simulink model "P2PHVDCMMC"  (R2024a)
settings: Solver=FixedStepDiscrete  StartTime=0.0  StopTime=10  RelTol=1e-3
PreLoadFcn:
  | % HVDCMMCInterconnectionParam
StartFcn:
  | tic
StopFcn:
  | toc
values from neighbouring files (symbols this model uses):
  C_PM = 1.758e-3    (= 0.001758)    [P2PHVDCMMCcode.m]    (also in SFu.mat)
  Cg = 50e-9    (= 5e-08)    [P2PHVDCMMCcode.m]    (also in SFu.mat)
  Fc = Fnom*3.37    (= 168.5)    [P2PHVDCMMCcode.m]    (also in SFu.mat)
  Fnom = 50    [P2PHVDCMMCcode.m]    (also in SFu.mat)
  HRM = 1    [SFu.mat]
  Ki_Ireg = 6    [P2PHVDCMMCcode.m]    (also in SFu.mat)
  Ki_Preg = 1.0    (= 1)    [P2PHVDCMMCcode.m]    (also in SFu.mat)
  Ki_Qreg = 1.0    (= 1)    [P2PHVDCMMCcode.m]    (also in SFu.mat)
  Ki_VDCreg = 100    [P2PHVDCMMCcode.m]    (also in SFu.mat)
  Kp_Ireg = 0.6    [P2PHVDCMMCcode.m]    (also in SFu.mat)
  Kp_Preg = 0.5/3    (= 0.166666666667)    [P2PHVDCMMCcode.m]    (also in SFu.mat)
  Kp_Qreg = 0.5/3    (= 0.166666666667)    [P2PHVDCMMCcode.m]    (also in SFu.mat)
  Kp_VDCreg = 4    [P2PHVDCMMCcode.m]    (also in SFu.mat)
  L_cable = 15e-3    (= 0.015)    [P2PHVDCMMCcode.m]    (also in SFu.mat)
  Larm = Larm_pu*(Zb_ac/(2*pi*Fnom))    [P2PHVDCMMCcode.m]    (also in SFu.mat = 0.0529455974536)
  Larm_pu = 0.15    [P2PHVDCMMCcode.m]    (also in SFu.mat)
  Lff = Larm_pu/2    (= 0.075)    [P2PHVDCMMCcode.m]    (also in SFu.mat)
  Limits_Ireg = [ 2.0  -2.0]    [P2PHVDCMMCcode.m]    (also in SFu.mat = [2 -2])
  Limits_Preg = [ 1.2, 0.8 ]    [P2PHVDCMMCcode.m]    (also in SFu.mat = [1.2 0.8])
  Limits_Qreg = [ 0.25, -0.25 ]    [P2PHVDCMMCcode.m]    (also in SFu.mat = [0.25 -0.25])
  Limits_VDCreg = [ 2.0  -2.0]    [P2PHVDCMMCcode.m]    (also in SFu.mat = [2 -2])
  Lxfo = 0.12    [P2PHVDCMMCcode.m]    (also in SFu.mat)
  N = 1    [P2PHVDCMMCcode.m]    (also in SFu.mat)
  Nb_PM = 36    [P2PHVDCMMCcode.m]    (also in SFu.mat)
  Pnom = 1000e6    (= 1000000000)    [P2PHVDCMMCcode.m]    (also in SFu.mat)
  R_cable = 0.5    [P2PHVDCMMCcode.m]    (also in SFu.mat)
  R_startup = 400    [P2PHVDCMMCcode.m]    (also in SFu.mat)
  Rarm = Rarm_pu*Zb_ac    [P2PHVDCMMCcode.m]    (also in SFu.mat = 0.1663335)
  Rff = Rarm_pu/2    (= 0.00075)    [P2PHVDCMMCcode.m]    (also in SFu.mat)
  Rg = 100    [P2PHVDCMMCcode.m]    (also in SFu.mat)
  Rxfo = 0.003    [P2PHVDCMMCcode.m]    (also in SFu.mat)
  S =     [SFu.mat]
  Slope_Qref = 0.5    [P2PHVDCMMCcode.m]    (also in SFu.mat)
  Slope_Vdc_ref = Vnom_dc/5    (= 128000)    [P2PHVDCMMCcode.m]    (also in SFu.mat)
  Tfault = 9999    [SFu.mat]
  Ts = Ts_Control    (= 4e-05)    [P2PHVDCMMCcode.m]    (also in SFu.mat)
  Ts_Control = 40e-6    (= 4e-05)    [P2PHVDCMMCcode.m]    (also in SFu.mat)
  Ts_dqn = 2e-5    (= 2e-05)    [P2PHVDCMMCcode.m]    (also in SFu.mat)
  Ts_Power = 20e-6    (= 2e-05)    [P2PHVDCMMCcode.m]    (also in SFu.mat)
  Vnom_dc = 640e3    (= 640000)    [P2PHVDCMMCcode.m]    (also in SFu.mat)
  Vnom_prim = 400e3    (= 400000)    [P2PHVDCMMCcode.m]    (also in SFu.mat)
  Vnom_sec = 333e3    (= 333000)    [P2PHVDCMMCcode.m]    (also in SFu.mat)
  Ws = 314.159265359    [SFu.mat]
undefined symbols (not defined in the file or in its folder): DiscIntNeverNeededParam, Discrete, DQN_Lib, gcbh, Int_DQNc_Mat, Mult_DQNc_Mat, Pcc, sps, sps_rtmsupport, spsMeanValueVariableFrequencyModel, spsPLL3phModel, SY3
libraries: simulink x38, spsControlledVoltageSourceLib x30, spsVoltageMeasurementLib x21, spsIdealSwitchLib x21, powerlib_extras x12, spsSecondOrderFilterLib x12, spsCurrentMeasurementLib x12, spsdq0toabcLib x9, spsMeanLib x8, spsMeanVariableFrequencyLib x8, spsabctodq0Lib x8, spsThreePhaseSeriesRLCBranchLib x7
(part 4 of 13)

== system P2PHVDCMMC/Controllers3/PLL, Measurements and Transformation ==
  note: P (pu) = Vd*Id + Vq*Iq
  note: Q (pu) = Vq*Id - Vd*Iq
  note: P positive = Converter generates active power (Inverter Mode)
  note: Q positive = Converter generates reactive power (Capacitive Mode)
  Vabc : Inport  PortDimensions=3
  Iabc : Inport  Port=2  PortDimensions=3
  Add : Sum  Inputs=1
  Demux : Demux  Outputs=2
  Discrete Mean value : powerlib_extras/Discrete Measurements/Discrete  Mean value  Freq=Fnom  Vinit=0  Ts=Ts
  Discrete Mean value1 : powerlib_extras/Discrete Measurements/Discrete  Mean value  Freq=Fnom  Vinit=0  Ts=Ts
  I->pu2 : Gain  Gain=sqrt(3)*Vnom_sec/sqrt(2)/Pnom  SaturateOnIntegerOverflow=on  OutDataTypeStr=Inherit: Same as input  ParamDataTypeStr=Inherit: Same as input
  PLL (3ph) : spsPLL3phLib/PLL (3ph)  Fmin=0.9*Fnom  Par_Init=[0, Fnom]  ParK=[180, 3200, 1]  TcD=1e-4  MaxRateChangeFreq=12  FilterCutOffFreq=25  Ts=Ts  AGC=on
  Product : Product  RndMeth=Zero
  Product1 : Product  RndMeth=Zero
  Second-Order Filter : spsSecondOrderFilterLib/Second-Order Filter  FilterType=Lowpass  Fo=Fn_filter  Zeta=Zeta_filter  Ts=Ts  Initialize=off  Vac_Init="[0,  0,  60]"  Vdc_Init=0  PlotResponse=off  FreqRange=[0, 500, 1]
  Second-Order Filter1 : spsSecondOrderFilterLib/Second-Order Filter  FilterType=Lowpass  Fo=Fn_filter  Zeta=Zeta_filter  Ts=Ts  Initialize=off  Vac_Init="[0,  0,  60]"  Vdc_Init=0  PlotResponse=off  FreqRange=[0, 500, 1]
  Selector3 : Selector  InputPortWidth=2  IndexOptions=Index vector (dialog)  Indices=[2 1]  OutputSizes=1
  Selector4 : Selector  InputPortWidth=3  IndexOptions=Index vector (dialog)  Indices=[1 2]  OutputSizes=1
  Selector5 : Selector  InputPortWidth=3  IndexOptions=Index vector (dialog)  Indices=[1 2]  OutputSizes=1
  Subtract : Sum  Inputs=+-
  V->pu1 : Gain  Gain=1/(Vnom_sec/sqrt(3)*sqrt(2))  SaturateOnIntegerOverflow=on  OutDataTypeStr=Inherit: Same as input  ParamDataTypeStr=Inherit: Same as input
  abc to dq0 : spsabctodq0Lib/abc to dq0  Alignment=90 degrees behind phase A axis
  abc to dq1 : spsabctodq0Lib/abc to dq0  Alignment=90 degrees behind phase A axis
  Freq : Outport
  wt : Outport  Port=2
  VdVq : Outport  Port=3
  IdIq : Outport  Port=4
  P : Outport  Port=5
  Q : Outport  Port=6
  wires:
  Selector3/1 -> Product1/1
  Discrete Mean value1/1 -> Q/1
  Discrete Mean value/1 -> P/1
  Second-Order Filter/1 -> VdVq/1, Product/1, Selector3/1
  Second-Order Filter1/1 -> IdIq/1, Product1/2, Product/2
  Product/1 -> Add/1
  Product1/1 -> Demux/1
  Demux/1 -> Subtract/1
  Demux/2 -> Subtract/2
  Add/1 -> Discrete Mean value/1
  Subtract/1 -> Discrete Mean value1/1
  abc to dq0/1 -> Selector4/1
  PLL (3ph)/1 -> Freq/1
  V->pu1/1 -> abc to dq0/1, PLL (3ph)/1
  Vabc/1 -> V->pu1/1
  PLL (3ph)/2 -> wt/1, abc to dq1/2, abc to dq0/2
  Iabc/1 -> I->pu2/1
  abc to dq1/1 -> Selector5/1
  I->pu2/1 -> abc to dq1/1
  Selector4/1 -> Second-Order Filter/1
  Selector5/1 -> Second-Order Filter1/1

== system P2PHVDCMMC/Controllers3/Reactive Power Regulator ==
  note: Reactive Power Regulator
  note: If PLL sync on Vprim --> Vq=0 --> Id = P/Vd et Iq = -1.0 * Q/Vd
  note: Q (pu) = Vq*Id - Vd*Iq (valid only for balanced & harmonics-free values)
  note: P (pu) = Vd*Id + Vq*Iq (Zero-sequence is not taken into account)
  VdVq_mes : Inport  PortDimensions=2
  Qmes : Inport  Port=2  PortDimensions=1
  Qref : Inport  Port=3  PortDimensions=1
  On : Inport  Port=4  PortDimensions=1
  Add2 : Sum
  Discrete Mean value1 : powerlib_extras/Discrete Measurements/Discrete  Mean value  Freq=Fnom  Vinit=0  Ts=Ts
  Discrete-Time Integrator : DiscreteIntegrator  SampleTime=Ts  LimitOutput=on  UpperSaturationLimit=Limits_Qreg(1)  LowerSaturationLimit=Limits_Qreg(2)  ICPrevOutput=DiscIntNeverNeededParam  ICPrevScaledInput=DiscIntNeverNeededParam
  Divide : Product  Inputs=*/
  Product : Product  RndMeth=Zero
  Product1 : Product  RndMeth=Zero
  Rtot_pu1 : Gain  Gain=-1  SaturateOnIntegerOverflow=on  OutDataTypeStr=Inherit: Same as input  ParamDataTypeStr=Inherit: Same as input
  Rtot_pu2 : Gain  Gain=-1  SaturateOnIntegerOverflow=on  OutDataTypeStr=Inherit: Same as input  ParamDataTypeStr=Inherit: Same as input
  Saturation : Saturate  UpperLimit=Limits_Qreg(1)  LowerLimit=Limits_Qreg(2)
  Saturation1 : Saturate  UpperLimit=2  LowerLimit=1e-6
  Saturation2 : Saturate  UpperLimit=Limits_Qreg(1)  LowerLimit=Limits_Qreg(2)
  Selector : Selector  InputPortWidth=2  IndexOptions=Index vector (dialog)  Indices=[1]  OutputSizes=1
  Sum : Sum  Inputs=|-+
  Sum6 : Sum  InputSameDT=on  SaturateOnIntegerOverflow=on  SampleTime=Ts  OutDataTypeStr=Inherit: Same as first input
  Switch1 : Switch  Criteria=u2 ~= 0  Threshold=0.5  OutDataTypeStr=double  SaturateOnIntegerOverflow=off  InputSameDT=off
  VdcNom_SM : Constant  Value=Kp_Qreg
  VdcNom_SM1 : Constant  Value=Ki_Qreg
  Zero-Order Hold : ZeroOrderHold  SampleTime=Ts
  Iq_ref : Outport
  wires:
  Saturation2/1 -> Rtot_pu1/1
  Saturation/1 -> Iq_ref/1
  Rtot_pu2/1 -> Add2/2
  Rtot_pu1/1 -> Add2/1
  Sum6/1 -> Saturation2/1
  Switch1/1 -> Product1/2, Product/2
  Sum/1 -> Switch1/1
  On/1 -> Switch1/2
  Add2/1 -> Saturation/1
  Product/1 -> Discrete-Time Integrator/1
  Product1/1 -> Zero-Order Hold/1
  VdcNom_SM/1 -> Product1/1
  VdcNom_SM1/1 -> Product/1
  Discrete-Time Integrator/1 -> Sum6/2
  Zero-Order Hold/1 -> Sum6/1
  Discrete Mean value1/1 -> Saturation1/1
  Saturation1/1 -> Divide/2
  Divide/1 -> Rtot_pu2/1
  Selector/1 -> Discrete Mean value1/1
  VdVq_mes/1 -> Selector/1
  Qmes/1 -> Sum/1
  Qref/1 -> Divide/1, Switch1/3, Sum/2

== system P2PHVDCMMC/DC & converter 2/Subsystem ==
  dcm1 : spsVoltageMeasurementLib/Voltage Measurement  PhasorSimulation=off  OutputType=Complex  PSBequivalent=0
  dcm2 : spsVoltageMeasurementLib/Voltage Measurement  PhasorSimulation=off  OutputType=Complex  PSBequivalent=0
  dcm3 : spsVoltageMeasurementLib/Voltage Measurement  PhasorSimulation=off  OutputType=Complex  PSBequivalent=0
  + : PMIOPort  Side=Left
  - : PMIOPort  Port=2  Side=Right
  tag scope: Vdc1=global, Vdc2=global, Vdc3=global
  wires:
  dcm3/1 -> [Vdc3]
  dcm2/1 -> [Vdc2]
  dcm1/1 -> [Vdc1]
  connections:
  dcm2/LConn1 -- dcm1/LConn1 -- +/RConn1 -- dcm3/LConn1
  dcm2/LConn2 -- -/RConn1 -- dcm3/LConn2 -- dcm1/LConn2

== system P2PHVDCMMC/MMC AVG_Inv/Circulating current suppression ==
  note: Circulating current Suppresion - Rectifier
  I_arm : Inport
  wt : Inport  Port=2
  Constant1 : Constant  Value=0
  Constant2 : Constant  Value=0
  Constant4 : Constant  Value=0
  Demux : Demux  Outputs=2
  Demux20 : Demux  Outputs=3
  Gain : Gain  Gain=0*Larm_pu
  Gain1 : Gain  Gain=0*Larm_pu
  Gain2 : Gain  Gain=-2
  Gain38 : Gain  Gain=1/2
  Gain39 : Gain  Gain=1/2
  Gain40 : Gain  Gain=1/2
  I->pu4 : Gain  Gain=sqrt(3)*Vnom_prim/sqrt(2)/Pnom  SaturateOnIntegerOverflow=on  OutDataTypeStr=Inherit: Same as input  ParamDataTypeStr=Inherit: Same as input
  Mux : Mux  Inputs=3
  Mux1 : Mux  Inputs=3
  PI regulator with anti-windup D : Subsystem  DialogController=POWERSYS.PowerSysDialog  mask(Discrete PI Controller){Kp=1, Ki=5, Par_Limits=Limits_Ireg, Init=0, Ts=Ts}
      mask prompts: Kp "Proportional gain (Kp):"; Ki "Integral gain (Ki):"; Par_Limits "Output limits: [ Upper   Lower ]"; Init "Output initial value:"; Ts "Sample time:"
      mask help: This block implements a discrete PI controller.
      mask init:
      | UpperLimit=Par_Limits(1);
      | LowerLimit=Par_Limits(2);
      | power_initmask();
      mask Help: This block is part of a subset of blocks in the Extras library that does not have documentation associated with it, other than the block mask description.
      mask Display: disp('PI');
  PI regulator with anti-windup D1 : Subsystem  DialogController=POWERSYS.PowerSysDialog  mask(Discrete PI Controller){Kp=1, Ki=5, Par_Limits=Limits_Ireg, Init=0, Ts=Ts}
      mask prompts: Kp "Proportional gain (Kp):"; Ki "Integral gain (Ki):"; Par_Limits "Output limits: [ Upper   Lower ]"; Init "Output initial value:"; Ts "Sample time:"
      mask help: This block implements a discrete PI controller.
      mask init:
      | UpperLimit=Par_Limits(1);
      | LowerLimit=Par_Limits(2);
      | power_initmask();
      mask Help: This block is part of a subset of blocks in the Extras library that does not have documentation associated with it, other than the block mask description.
      mask Display: disp('PI');
  Rate Transition1 : RateTransition  OutPortSampleTime=Ts_Control
  Rate Transition8 : RateTransition  OutPortSampleTime=Ts_Control
  Saturation1 : Saturate  UpperLimit=2  LowerLimit=-2
  Scope : Scope
  Scope1 : Scope
  Selector : Selector  InputPortWidth=3  IndexOptions=Index vector (dialog)  Indices=[1 2]  OutputSizes=1
  Sum1 : Sum  Inputs=-+|
  Sum2 : Sum  Inputs=|+-
  Sum78 : Sum  Inputs=|++
  Sum80 : Sum  Inputs=+
  Sum81 : Sum  Inputs=+
  Sum82 : Sum  Inputs=+
  Sum83 : Sum  Inputs=-+|
  Sum85 : Sum  Inputs=|+-
  abc to dq0 : spsabctodq0Lib/abc to dq0  Alignment=90 degrees behind phase A axis
  dq0 to abc : spsdq0toabcLib/dq0 to abc  Alignment=90 degrees behind phase A axis
  V_diffi : Outport  VectorParamsAs1DForOutWhenUnconnected=off
  wires:
  Saturation1/1 -> V_diffi/1
  Gain40/1 -> Mux/3
  Demux20/2 -> Sum81/1
  Constant2/1 -> Sum85/1
  Constant4/1 -> Mux1/3
  Sum1/1 -> Mux1/2
  PI regulator with anti-windup D1/1(Out) -> Sum1/2
  PI regulator with anti-windup D/1(Out) -> Sum78/1
  Mux1/1 -> dq0 to abc/1
  Selector/1 -> Scope1/1, Demux/1
  Gain/1 -> Sum1/1
  Sum78/1 -> Mux1/1
  Demux20/3 -> Sum82/1
  Sum85/1 -> PI regulator with anti-windup D/1(Error)
  abc to dq0/1 -> Selector/1
  Demux20/1 -> Sum80/1
  I->pu4/1 -> Rate Transition8/1
  Rate Transition8/1 -> Demux20/1
  Sum80/1 -> Gain38/1
  Sum83/1 -> PI regulator with anti-windup D1/1(Error)
  Constant1/1 -> Sum83/2
  Gain39/1 -> Mux/2
  Sum81/1 -> Gain39/1
  Sum82/1 -> Gain40/1
  dq0 to abc/1 -> Saturation1/1
  Demux/2 -> Sum83/1, Gain1/1
  Gain1/1 -> Sum78/2
  Demux/1 -> Sum85/2, Gain/1
  Gain38/1 -> Mux/1
  wt/1 -> Gain2/1
  Gain2/1 -> dq0 to abc/2, abc to dq0/2
  I_arm/1 -> I->pu4/1
  Mux/1 -> abc to dq0/1, Sum2/1
  Sum2/1 -> Scope/1
  [Isec] -> Rate Transition1/1
  Rate Transition1/1 -> Sum2/2

== system P2PHVDCMMC/MMC AVG_Inv/SB1 ==
  CT1 : spsCurrentMeasurementLib/Current Measurement  PhasorSimulation=off  OutputType=Complex  PSBequivalent=0
  Goto19 : Goto  Commented=on  GotoTag=V12_Ap  TagVisibility=global
  Voltage Measurement : spsVoltageMeasurementLib/Voltage Measurement  Commented=on  PhasorSimulation=off  OutputType=Complex  PSBequivalent=0
  I1 : PMIOPort  Side=Left
  I2 : PMIOPort  Port=2  Side=Left
  O1 : PMIOPort  Port=3  Side=Right
  O2 : PMIOPort  Port=4  Side=Right
  tag scope: ITa_inv=global
  wires:
  CT1/1 -> [ITa_inv]
  Voltage Measurement/1 -> Goto19/1
  connections:
  CT1/RConn1 -- Voltage Measurement/LConn1 -- I1/RConn1
  CT1/LConn1 -- O1/RConn1
  I2/RConn1 -- Voltage Measurement/LConn2 -- O2/RConn1

== system P2PHVDCMMC/MMC AVG_Inv/SB2 ==
  CT2 : spsCurrentMeasurementLib/Current Measurement  PhasorSimulation=off  OutputType=Complex  PSBequivalent=0
  Goto19 : Goto  Commented=on  GotoTag=V12_Bp  TagVisibility=global
  Voltage Measurement : spsVoltageMeasurementLib/Voltage Measurement  Commented=on  PhasorSimulation=off  OutputType=Complex  PSBequivalent=0
  I1 : PMIOPort  Side=Left
  I2 : PMIOPort  Port=2  Side=Left
  O1 : PMIOPort  Port=3  Side=Right
  O2 : PMIOPort  Port=4  Side=Right
  tag scope: ITb_inv=global
  wires:
  Voltage Measurement/1 -> Goto19/1
  CT2/1 -> [ITb_inv]
  connections:
  Voltage Measurement/LConn2 -- O2/RConn1 -- I2/RConn1
  CT2/LConn1 -- O1/RConn1
  Voltage Measurement/LConn1 -- CT2/RConn1 -- I1/RConn1

== system P2PHVDCMMC/MMC AVG_Inv/SB3 ==
  CT3 : spsCurrentMeasurementLib/Current Measurement  PhasorSimulation=off  OutputType=Complex  PSBequivalent=0
  Goto19 : Goto  Commented=on  GotoTag=V12_Cp  TagVisibility=global
  Voltage Measurement : spsVoltageMeasurementLib/Voltage Measurement  Commented=on  PhasorSimulation=off  OutputType=Complex  PSBequivalent=0
  I1 : PMIOPort  Side=Left
  I2 : PMIOPort  Port=2  Side=Left
  O1 : PMIOPort  Port=3  Side=Right
  O2 : PMIOPort  Port=4  Side=Right
  tag scope: ITc_inv=global
  wires:
  CT3/1 -> [ITc_inv]
  Voltage Measurement/1 -> Goto19/1
  connections:
  I1/RConn1 -- CT3/RConn1 -- Voltage Measurement/LConn1
  CT3/LConn1 -- O1/RConn1
  I2/RConn1 -- O2/RConn1 -- Voltage Measurement/LConn2

== system P2PHVDCMMC/MMC AVG_Inv/SB4 ==
  CT4 : spsCurrentMeasurementLib/Current Measurement  PhasorSimulation=off  OutputType=Complex  PSBequivalent=0
  Goto19 : Goto  Commented=on  GotoTag=V12_Am  TagVisibility=global
  Voltage Measurement : spsVoltageMeasurementLib/Voltage Measurement  Commented=on  PhasorSimulation=off  OutputType=Complex  PSBequivalent=0
  I1 : PMIOPort  Side=Left
  I2 : PMIOPort  Port=2  Side=Left
  O1 : PMIOPort  Port=3  Side=Right
  O2 : PMIOPort  Port=4  Side=Right
  tag scope: IBa_inv=global
  wires:
  Voltage Measurement/1 -> Goto19/1
  CT4/1 -> [IBa_inv]
  connections:
  Voltage Measurement/LConn2 -- O2/RConn1 -- I2/RConn1
  CT4/LConn1 -- O1/RConn1
  Voltage Measurement/LConn1 -- CT4/RConn1 -- I1/RConn1

== system P2PHVDCMMC/MMC AVG_Inv/SB5 ==
  CT5 : spsCurrentMeasurementLib/Current Measurement  PhasorSimulation=off  OutputType=Complex  PSBequivalent=0
  Goto19 : Goto  Commented=on  GotoTag=V12_Bm  TagVisibility=global
  Voltage Measurement : spsVoltageMeasurementLib/Voltage Measurement  Commented=on  PhasorSimulation=off  OutputType=Complex  PSBequivalent=0
  I1 : PMIOPort  Side=Left
  I2 : PMIOPort  Port=2  Side=Left
  O1 : PMIOPort  Port=3  Side=Right
  O2 : PMIOPort  Port=4  Side=Right
  tag scope: IBb_inv=global
  wires:
  CT5/1 -> [IBb_inv]
  Voltage Measurement/1 -> Goto19/1
  connections:
  I1/RConn1 -- CT5/RConn1 -- Voltage Measurement/LConn1
  CT5/LConn1 -- O1/RConn1
  I2/RConn1 -- O2/RConn1 -- Voltage Measurement/LConn2

== system P2PHVDCMMC/MMC AVG_Inv/SB6 ==
  CT6 : spsCurrentMeasurementLib/Current Measurement  PhasorSimulation=off  OutputType=Complex  PSBequivalent=0
  Goto19 : Goto  Commented=on  GotoTag=V12_Cm  TagVisibility=global
  Voltage Measurement : spsVoltageMeasurementLib/Voltage Measurement  Commented=on  PhasorSimulation=off  OutputType=Complex  PSBequivalent=0
  I1 : PMIOPort  Side=Left
  I2 : PMIOPort  Port=2  Side=Left
  O1 : PMIOPort  Port=3  Side=Right
  O2 : PMIOPort  Port=4  Side=Right
  tag scope: IBc_inv=global
  wires:
  Voltage Measurement/1 -> Goto19/1
  CT6/1 -> [IBc_inv]
  connections:
  Voltage Measurement/LConn2 -- O2/RConn1 -- I2/RConn1
  CT6/LConn1 -- O1/RConn1
  Voltage Measurement/LConn1 -- CT6/RConn1 -- I1/RConn1

== system P2PHVDCMMC/MMC AVG_Inv/Subsystem3 ==
  Demux3 : Demux  Commented=on  Outputs=3
  From13 : From  Commented=on  GotoTag=IBa  TagVisibility=global
  From22 : From  Commented=on  GotoTag=Isec  TagVisibility=global
  From25 : From  Commented=on  GotoTag=Converter2_On  TagVisibility=global
  From9 : From  Commented=on  GotoTag=ITa  TagVisibility=global
  Gain : Gain  Commented=on  Gain=1/2
  Scope : Scope  Commented=on  NumInputPorts=2
  Subsystem : Subsystem  Commented=on
      settings: PortSchema="{\"entries\":[{\"content\":{\"sides\":[{\"content\":{\"connectorIds\":[\"In1\"]},\"type\":\"ConnectorPlacement.EquallySpacedRectSide\",\"uuid\":\"6a070030-9d36-4614-a6ed-5c0106204a15\"},{\"content\":{\"side\":\"RIGHT\"},\"type\":\"ConnectorPlacement.EquallySpacedRectSide\",\"uuid\":\"80e8cce1-ebd9-4d3c-9a33-26e83fa71e17\"},{\"content\":{\"connectorIds\":[\"LConn1\",\"LConn2\",\"LConn3\"],\"side\":\"TOP\"},\"type\":\"ConnectorPlacement.EquallySpacedRectSide\",\"uuid\":\"873c34e2-09cd-4b1f-a733-63c02c066783\"},{\"content\":{\"connectorIds\":[\"RConn1\",\"RConn2\",\"RConn3\"],\"side\":\"BOTTOM\"},\"type\":\"ConnectorPlacement.EquallySpacedRectSide\",\"uuid\":\"2e3fd9e5-67ce-4b4a-a343-b8208a9902db\"}]},\"type\":\"ConnectorPlacement.EquallySpacedConnector\",\"uuid\":\"0790a5cd-c0d6-472f-8eb5-e46769681968\"}],\"packageUris\":[\"http://schema.mathworks.com/mf0/Connector/R2020b\"],\"version\":\"1.0\"}"
  Subsystem1 : Subsystem  Commented=on
      settings: PortSchema="{\"entries\":[{\"content\":{\"sides\":[{\"content\":{\"connectorIds\":[\"In1\"]},\"type\":\"ConnectorPlacement.EquallySpacedRectSide\",\"uuid\":\"a5cee0a7-b338-4dc7-83bc-48872831f323\"},{\"content\":{\"side\":\"RIGHT\"},\"type\":\"ConnectorPlacement.EquallySpacedRectSide\",\"uuid\":\"ca317b42-2c00-457f-a5f3-7770b49527a9\"},{\"content\":{\"connectorIds\":[\"LConn1\",\"LConn2\",\"LConn3\"],\"side\":\"TOP\"},\"type\":\"ConnectorPlacement.EquallySpacedRectSide\",\"uuid\":\"77de2851-5038-4e86-9464-a1f28ff8b83a\"},{\"content\":{\"connectorIds\":[\"RConn1\",\"RConn2\",\"RConn3\"],\"side\":\"BOTTOM\"},\"type\":\"ConnectorPlacement.EquallySpacedRectSide\",\"uuid\":\"3c356faa-cb69-49bf-bf76-45ac18baf20f\"}]},\"type\":\"ConnectorPlacement.EquallySpacedConnector\",\"uuid\":\"03d4a433-e9ae-4343-977e-c6031a8cb266\"}],\"packageUris\":[\"http://schema.mathworks.com/mf0/Connector/R2020b\"],\"version\":\"1.0\"}"
  Subsystem2 : Subsystem  Commented=on
      settings: PortSchema="{\"entries\":[{\"content\":{\"sides\":[{\"content\":{\"connectorIds\":[\"In1\"]},\"type\":\"ConnectorPlacement.EquallySpacedRectSide\",\"uuid\":\"a5cee0a7-b338-4dc7-83bc-48872831f323\"},{\"content\":{\"side\":\"RIGHT\"},\"type\":\"ConnectorPlacement.EquallySpacedRectSide\",\"uuid\":\"ca317b42-2c00-457f-a5f3-7770b49527a9\"},{\"content\":{\"connectorIds\":[\"LConn1\",\"LConn2\",\"LConn3\"],\"side\":\"TOP\"},\"type\":\"ConnectorPlacement.EquallySpacedRectSide\",\"uuid\":\"77de2851-5038-4e86-9464-a1f28ff8b83a\"},{\"content\":{\"connectorIds\":[\"RConn1\",\"RConn2\",\"RConn3\"],\"side\":\"BOTTOM\"},\"type\":\"ConnectorPlacement.EquallySpacedRectSide\",\"uuid\":\"3c356faa-cb69-49bf-bf76-45ac18baf20f\"}]},\"type\":\"ConnectorPlacement.EquallySpacedConnector\",\"uuid\":\"03d4a433-e9ae-4343-977e-c6031a8cb266\"}],\"packageUris\":[\"http://schema.mathworks.com/mf0/Connector/R2020b\"],\"version\":\"1.0\"}"
  Sum : Sum  Commented=on  Inputs=|++
  Sum1 : Sum  Commented=on  Inputs=|+-
  1 : PMIOPort  Side=Left
  2 : PMIOPort  Port=2  Side=Left
  3 : PMIOPort  Port=3  Side=Left
  5 : PMIOPort  Port=4  Side=Right
  4 : PMIOPort  Port=5  Side=Right
  6 : PMIOPort  Port=6  Side=Right
  7 : PMIOPort  Port=7  Side=Right
  8 : PMIOPort  Port=8  Side=Right
  Out1 : Outport
  Out2 : Outport  Port=2
  wires:
  Sum1/1 -> Scope/2
  From22/1 -> Demux3/1
  Gain/1 -> Sum1/1, Scope/1
  Demux3/1 -> Sum1/2
  Sum/1 -> Gain/1
  From13/1 -> Sum/2
  From25/1 -> Subsystem2/1(g), Subsystem1/1(g)
  From9/1 -> Sum/1
  Demux3/2 -> Out1/1
  Demux3/3 -> Out2/1
  connections:
  Subsystem1/LConn3 -- 3/RConn1
  Subsystem2/LConn1 -- 4/RConn1 -- Subsystem2/LConn3 -- Subsystem2/LConn2
  Subsystem1/RConn3 -- 5/RConn1 -- Subsystem1/RConn1 -- Subsystem1/RConn2
  Subsystem2/RConn1 -- 6/RConn1
  Subsystem2/RConn2 -- 7/RConn1
  Subsystem2/RConn3 -- 8/RConn1
  Subsystem1/LConn1 -- 1/RConn1
  Subsystem1/LConn2 -- 2/RConn1

== system P2PHVDCMMC/MMC AVG_Rec/Circulating current suppression ==
  note: Circulating current Suppresion - Rectifier
  I_arm : Inport
  wt : Inport  Port=2
  Constant1 : Constant  Value=0
  Constant2 : Constant  Value=0
  Constant4 : Constant  Value=0
  Demux : Demux  Outputs=2
  Demux20 : Demux  Outputs=3
  Gain : Gain  Gain=0*Larm_pu
  Gain1 : Gain  Gain=0*Larm_pu
  Gain2 : Gain  Gain=-2
  Gain38 : Gain  Gain=1/2
  Gain39 : Gain  Gain=1/2
  Gain40 : Gain  Gain=1/2
  I->pu4 : Gain  Gain=sqrt(3)*Vnom_prim/sqrt(2)/Pnom  SaturateOnIntegerOverflow=on  OutDataTypeStr=Inherit: Same as input  ParamDataTypeStr=Inherit: Same as input
  Mux : Mux  Inputs=3
  Mux1 : Mux  Inputs=3
  PI regulator with anti-windup D : Subsystem  DialogController=POWERSYS.PowerSysDialog  mask(Discrete PI Controller){Kp=1, Ki=5, Par_Limits=Limits_Ireg, Init=0, Ts=Ts}
      mask prompts: Kp "Proportional gain (Kp):"; Ki "Integral gain (Ki):"; Par_Limits "Output limits: [ Upper   Lower ]"; Init "Output initial value:"; Ts "Sample time:"
      mask help: This block implements a discrete PI controller.
      mask init:
      | UpperLimit=Par_Limits(1);
      | LowerLimit=Par_Limits(2);
      | power_initmask();
      mask Help: This block is part of a subset of blocks in the Extras library that does not have documentation associated with it, other than the block mask description.
      mask Display: disp('PI');
  PI regulator with anti-windup D1 : Subsystem  DialogController=POWERSYS.PowerSysDialog  mask(Discrete PI Controller){Kp=1, Ki=5, Par_Limits=Limits_Ireg, Init=0, Ts=Ts}
      mask prompts: Kp "Proportional gain (Kp):"; Ki "Integral gain (Ki):"; Par_Limits "Output limits: [ Upper   Lower ]"; Init "Output initial value:"; Ts "Sample time:"
      mask help: This block implements a discrete PI controller.
      mask init:
      | UpperLimit=Par_Limits(1);
      | LowerLimit=Par_Limits(2);
      | power_initmask();
      mask Help: This block is part of a subset of blocks in the Extras library that does not have documentation associated with it, other than the block mask description.
      mask Display: disp('PI');
  Rate Transition1 : RateTransition  OutPortSampleTime=Ts_Control
  Rate Transition8 : RateTransition  OutPortSampleTime=Ts_Control
  Saturation1 : Saturate  UpperLimit=2  LowerLimit=-2
  Scope : Scope  Commented=on
  Scope1 : Scope  Commented=on
  Selector : Selector  InputPortWidth=3  IndexOptions=Index vector (dialog)  Indices=[1 2]  OutputSizes=1
  Sum1 : Sum  Inputs=-+|
  Sum2 : Sum  Inputs=|+-
  Sum78 : Sum  Inputs=|++
  Sum80 : Sum  Inputs=+
  Sum81 : Sum  Inputs=+
  Sum82 : Sum  Inputs=+
  Sum83 : Sum  Inputs=-+|
  Sum85 : Sum  Inputs=|+-
  abc to dq0 : spsabctodq0Lib/abc to dq0  Alignment=90 degrees behind phase A axis
  dq0 to abc : spsdq0toabcLib/dq0 to abc  Alignment=90 degrees behind phase A axis
  V_diffi : Outport  VectorParamsAs1DForOutWhenUnconnected=off
  wires:
  Saturation1/1 -> V_diffi/1
  Gain40/1 -> Mux/3
  Demux20/2 -> Sum81/1
  Constant2/1 -> Sum85/1
  Constant4/1 -> Mux1/3
  Sum1/1 -> Mux1/2
  PI regulator with anti-windup D1/1(Out) -> Sum1/2
  PI regulator with anti-windup D/1(Out) -> Sum78/1
  Mux1/1 -> dq0 to abc/1
  Selector/1 -> Scope1/1, Demux/1
  Gain/1 -> Sum1/1
  Sum78/1 -> Mux1/1
  Demux20/3 -> Sum82/1
  Sum85/1 -> PI regulator with anti-windup D/1(Error)
  abc to dq0/1 -> Selector/1
  Demux20/1 -> Sum80/1
  I->pu4/1 -> Rate Transition8/1
  Rate Transition8/1 -> Demux20/1
  Sum80/1 -> Gain38/1
  Sum83/1 -> PI regulator with anti-windup D1/1(Error)
  Constant1/1 -> Sum83/2
  Gain39/1 -> Mux/2
  Sum81/1 -> Gain39/1
  Sum82/1 -> Gain40/1
  dq0 to abc/1 -> Saturation1/1
  Demux/2 -> Sum83/1, Gain1/1
  Gain1/1 -> Sum78/2
  Demux/1 -> Sum85/2, Gain/1
  Gain38/1 -> Mux/1
  wt/1 -> Gain2/1
  Gain2/1 -> dq0 to abc/2, abc to dq0/2
  I_arm/1 -> I->pu4/1
  Mux/1 -> abc to dq0/1, Sum2/1
  Sum2/1 -> Scope/1
  [Isec] -> Rate Transition1/1
  Rate Transition1/1 -> Sum2/2

== system P2PHVDCMMC/MMC AVG_Rec/SB1 ==
  CT1 : spsCurrentMeasurementLib/Current Measurement  PhasorSimulation=off  OutputType=Complex  PSBequivalent=0
  Goto19 : Goto  Commented=on  GotoTag=V12_Ap  TagVisibility=global
  Voltage Measurement : spsVoltageMeasurementLib/Voltage Measurement  Commented=on  PhasorSimulation=off  OutputType=Complex  PSBequivalent=0
  I1 : PMIOPort  Side=Left
  I2 : PMIOPort  Port=2  Side=Left
  O1 : PMIOPort  Port=3  Side=Right
  O2 : PMIOPort  Port=4  Side=Right
  tag scope: ITa=global
  wires:
  CT1/1 -> [ITa]
  Voltage Measurement/1 -> Goto19/1
  connections:
  CT1/RConn1 -- Voltage Measurement/LConn1 -- I1/RConn1
  CT1/LConn1 -- O1/RConn1
  I2/RConn1 -- Voltage Measurement/LConn2 -- O2/RConn1

== system P2PHVDCMMC/MMC AVG_Rec/SB2 ==
  CT2 : spsCurrentMeasurementLib/Current Measurement  PhasorSimulation=off  OutputType=Complex  PSBequivalent=0
  Goto19 : Goto  Commented=on  GotoTag=V12_Bp  TagVisibility=global
  Voltage Measurement : spsVoltageMeasurementLib/Voltage Measurement  Commented=on  PhasorSimulation=off  OutputType=Complex  PSBequivalent=0
  I1 : PMIOPort  Side=Left
  I2 : PMIOPort  Port=2  Side=Left
  O1 : PMIOPort  Port=3  Side=Right
  O2 : PMIOPort  Port=4  Side=Right
  tag scope: ITb=global
  wires:
  Voltage Measurement/1 -> Goto19/1
  CT2/1 -> [ITb]
  connections:
  Voltage Measurement/LConn2 -- O2/RConn1 -- I2/RConn1
  CT2/LConn1 -- O1/RConn1
  Voltage Measurement/LConn1 -- CT2/RConn1 -- I1/RConn1

== system P2PHVDCMMC/MMC AVG_Rec/SB3 ==
  CT3 : spsCurrentMeasurementLib/Current Measurement  PhasorSimulation=off  OutputType=Complex  PSBequivalent=0
  Goto19 : Goto  Commented=on  GotoTag=V12_Cp  TagVisibility=global
  Voltage Measurement : spsVoltageMeasurementLib/Voltage Measurement  Commented=on  PhasorSimulation=off  OutputType=Complex  PSBequivalent=0
  I1 : PMIOPort  Side=Left
  I2 : PMIOPort  Port=2  Side=Left
  O1 : PMIOPort  Port=3  Side=Right
  O2 : PMIOPort  Port=4  Side=Right
  tag scope: ITc=global
  wires:
  CT3/1 -> [ITc]
  Voltage Measurement/1 -> Goto19/1
  connections:
  I1/RConn1 -- CT3/RConn1 -- Voltage Measurement/LConn1
  CT3/LConn1 -- O1/RConn1
  I2/RConn1 -- O2/RConn1 -- Voltage Measurement/LConn2

== system P2PHVDCMMC/MMC AVG_Rec/SB4 ==
  CT4 : spsCurrentMeasurementLib/Current Measurement  PhasorSimulation=off  OutputType=Complex  PSBequivalent=0
  Goto19 : Goto  Commented=on  GotoTag=V12_Am  TagVisibility=global
  Voltage Measurement : spsVoltageMeasurementLib/Voltage Measurement  Commented=on  PhasorSimulation=off  OutputType=Complex  PSBequivalent=0
  I1 : PMIOPort  Side=Left
  I2 : PMIOPort  Port=2  Side=Left
  O1 : PMIOPort  Port=3  Side=Right
  O2 : PMIOPort  Port=4  Side=Right
  tag scope: IBa=global
  wires:
  Voltage Measurement/1 -> Goto19/1
  CT4/1 -> [IBa]
  connections:
  Voltage Measurement/LConn2 -- O2/RConn1 -- I2/RConn1
  CT4/LConn1 -- O1/RConn1
  Voltage Measurement/LConn1 -- CT4/RConn1 -- I1/RConn1

== system P2PHVDCMMC/MMC AVG_Rec/SB5 ==
  CT5 : spsCurrentMeasurementLib/Current Measurement  PhasorSimulation=off  OutputType=Complex  PSBequivalent=0
  Goto19 : Goto  Commented=on  GotoTag=V12_Bm  TagVisibility=global
  Voltage Measurement : spsVoltageMeasurementLib/Voltage Measurement  Commented=on  PhasorSimulation=off  OutputType=Complex  PSBequivalent=0
  I1 : PMIOPort  Side=Left
  I2 : PMIOPort  Port=2  Side=Left
  O1 : PMIOPort  Port=3  Side=Right
  O2 : PMIOPort  Port=4  Side=Right
  tag scope: IBb=global
  wires:
  CT5/1 -> [IBb]
  Voltage Measurement/1 -> Goto19/1
  connections:
  I1/RConn1 -- CT5/RConn1 -- Voltage Measurement/LConn1
  CT5/LConn1 -- O1/RConn1
  I2/RConn1 -- O2/RConn1 -- Voltage Measurement/LConn2

== system P2PHVDCMMC/MMC AVG_Rec/SB6 ==
  CT6 : spsCurrentMeasurementLib/Current Measurement  PhasorSimulation=off  OutputType=Complex  PSBequivalent=0
  Goto19 : Goto  Commented=on  GotoTag=V12_Cm  TagVisibility=global
  Voltage Measurement : spsVoltageMeasurementLib/Voltage Measurement  Commented=on  PhasorSimulation=off  OutputType=Complex  PSBequivalent=0
  I1 : PMIOPort  Side=Left
  I2 : PMIOPort  Port=2  Side=Left
  O1 : PMIOPort  Port=3  Side=Right
  O2 : PMIOPort  Port=4  Side=Right
  tag scope: IBc=global
  wires:
  Voltage Measurement/1 -> Goto19/1
  CT6/1 -> [IBc]
  connections:
  Voltage Measurement/LConn2 -- O2/RConn1 -- I2/RConn1
  CT6/LConn1 -- O1/RConn1
  Voltage Measurement/LConn1 -- CT6/RConn1 -- I1/RConn1

== system P2PHVDCMMC/MMC AVG_Rec/Subsystem1 ==
  wt : Inport
  Circulating current suppression1 : Subsystem  Commented=on  VariantControl=Variant1
  Constant3 : Constant  Commented=on  Value="complex([[0 1; 0  0; 0 0 ],[zeros(3,N+2)]])"
  Demux3 : Demux  Commented=on  Outputs=3
  From13 : From  Commented=on  GotoTag=IBa  TagVisibility=global
  From22 : From  Commented=on  GotoTag=Isec  TagVisibility=global
  From24 : From  Commented=on  GotoTag=Converter2_On  TagVisibility=global
  From25 : From  Commented=on  GotoTag=Iup
  From35 : From  Commented=on  GotoTag=Ilow
  From9 : From  Commented=on  GotoTag=ITa  TagVisibility=global
  Gain : Gain  Commented=on  Gain=1/2
  Rate Transition2 : RateTransition  Commented=on  OutPortSampleTime=Ts_Power
  Scope : Scope  Commented=on  NumInputPorts=2
  Subsystem : Subsystem  Commented=on
      settings: PortSchema="{\"entries\":[{\"content\":{\"sides\":[{\"content\":{\"connectorIds\":[\"In1\"]},\"type\":\"ConnectorPlacement.EquallySpacedRectSide\",\"uuid\":\"6a070030-9d36-4614-a6ed-5c0106204a15\"},{\"content\":{\"side\":\"RIGHT\"},\"type\":\"ConnectorPlacement.EquallySpacedRectSide\",\"uuid\":\"80e8cce1-ebd9-4d3c-9a33-26e83fa71e17\"},{\"content\":{\"connectorIds\":[\"LConn1\",\"LConn2\",\"LConn3\"],\"side\":\"TOP\"},\"type\":\"ConnectorPlacement.EquallySpacedRectSide\",\"uuid\":\"873c34e2-09cd-4b1f-a733-63c02c066783\"},{\"content\":{\"connectorIds\":[\"RConn1\",\"RConn2\",\"RConn3\"],\"side\":\"BOTTOM\"},\"type\":\"ConnectorPlacement.EquallySpacedRectSide\",\"uuid\":\"2e3fd9e5-67ce-4b4a-a343-b8208a9902db\"}]},\"type\":\"ConnectorPlacement.EquallySpacedConnector\",\"uuid\":\"0790a5cd-c0d6-472f-8eb5-e46769681968\"}],\"packageUris\":[\"http://schema.mathworks.com/mf0/Connector/R2020b\"],\"version\":\"1.0\"}"
  Sum : Sum  Commented=on  Inputs=|++
  Sum1 : Sum  Commented=on  Inputs=|+-
  Sum2 : Sum  Commented=on  Inputs=|++
  + : PMIOPort  Side=Left
  +3 : PMIOPort  Port=2  Side=Left
  +1 : PMIOPort  Port=3  Side=Left
  - : PMIOPort  Port=4  Side=Right
  -1 : PMIOPort  Port=5  Side=Right
  -2 : PMIOPort  Port=6  Side=Right
  Out1 : Outport
  Out2 : Outport  Port=2
  Out3 : Outport  Port=3
  wires:
  Demux3/1 -> Sum1/2
  From22/1 -> Demux3/1
  From25/1 -> Sum2/1
  From24/1 -> Subsystem/1(g)
  Sum1/1 -> Scope/2
  Gain/1 -> Sum1/1, Scope/1
  From13/1 -> Sum/2
  Sum/1 -> Gain/1
  From9/1 -> Sum/1
  Circulating current suppression1/1(V_diffi) -> Rate Transition2/1  "Mac_EMT"
  From35/1 -> Sum2/2
  Sum2/1 -> Circulating current suppression1/1(I_arm)
  Rate Transition2/1 -> Out1/1
  wt/1 -> Circulating current suppression1/2(wt)
  Demux3/2 -> Out2/1
  Demux3/3 -> Out3/1
  connections:
  Subsystem/LConn1 -- +/RConn1
  Subsystem/LConn3 -- +3/RConn1
  Subsystem/RConn2 -- -1/RConn1
  Subsystem/RConn1 -- -/RConn1
  Subsystem/LConn2 -- +1/RConn1
  Subsystem/RConn3 -- -2/RConn1

== system P2PHVDCMMC/Subsystem4/ACinv ==
  Add3 : Sum
  Add4 : Sum
  Circulating current suppression2 : Subsystem  VariantControl=Variant1
  Constant14 : Constant  Value="complex([[0 0; 0  0; 1 0 ],[zeros(3,N+2)]])"
  Constant16 : Constant  Value="complex([[0 0; 0  0; 1 0 ],[zeros(3,N+2)]])"
  Gain1 : Gain  Gain=1/(C_PM / Nb_PM)
  Gain15 : Gain  Gain=0.5
  Gain4 : Gain  Gain=-1
  Gain6 : Gain  Gain=0.5
  Gain7 : Gain  Gain=1/(C_PM / Nb_PM)
  Int_DQNc_Mat1 : MATLAB Function  AncestorBlock=DQN_Lib/Int_DQNc_Mat  TreatAsAtomicUnit=on  SystemSampleTime=Ts_dqn  mask{N=7+N, dt=2e-5, w=Ws, InitInt=0*[0.8; 0.6; -0.33], swFeed=off, R=1, iL=1}
      mask prompts: N "Order number:"; dt "Time step (s):"; w "Angular frequency (1/rad):"; InitInt "Initial conditions DC [3x1]:"; swFeed "Enable feedback"; R "Feedback parameter (Kr {abc}):"; iL "Feedback parameter (Ki {abc}):"
  Int_DQNc_Mat2 : MATLAB Function  AncestorBlock=DQN_Lib/Int_DQNc_Mat  TreatAsAtomicUnit=on  SystemSampleTime=Ts_dqn  mask{N=7+N, dt=2e-5, w=Ws, InitInt=0*[0.8; 0.6; -0.33], swFeed=off, R=1, iL=1}
      mask prompts: N "Order number:"; dt "Time step (s):"; w "Angular frequency (1/rad):"; InitInt "Initial conditions DC [3x1]:"; swFeed "Enable feedback"; R "Feedback parameter (Kr {abc}):"; iL "Feedback parameter (Ki {abc}):"
  Mult_DQNc_Mat1 : MATLAB Function  AncestorBlock=DQN_Lib/Mult_DQNc_Mat  TreatAsAtomicUnit=on  SystemSampleTime=Ts_dqn  mask{N=7+N, HrmDbl=on}
      mask prompts: N "Harmonic order:"; HrmDbl "Double Harmonic"
  Mult_DQNc_Mat2 : MATLAB Function  AncestorBlock=DQN_Lib/Mult_DQNc_Mat  TreatAsAtomicUnit=on  SystemSampleTime=Ts_dqn  mask{N=7+N, HrmDbl=on}
      mask prompts: N "Harmonic order:"; HrmDbl "Double Harmonic"
  Mult_DQNc_Mat3 : MATLAB Function  AncestorBlock=DQN_Lib/Mult_DQNc_Mat  TreatAsAtomicUnit=on  SystemSampleTime=Ts_dqn  mask{N=3+N, HrmDbl=on}
      mask prompts: N "Harmonic order:"; HrmDbl "Double Harmonic"
  Mult_DQNc_Mat4 : MATLAB Function  AncestorBlock=DQN_Lib/Mult_DQNc_Mat  TreatAsAtomicUnit=on  SystemSampleTime=Ts_dqn  mask{N=3+N, HrmDbl=on}
      mask prompts: N "Harmonic order:"; HrmDbl "Double Harmonic"
  Mux13 : Concatenate  Mode=Multidimensional array
  Selector10 : Selector  NumberOfDimensions=2  InputPortWidth=size(SY3.C,1)  IndexOptions=Select all,Index vector (dialog)  Indices=4:6,1:[N+4]  OutputSizes=1,1
  Selector11 : Selector  NumberOfDimensions=2  InputPortWidth=size(SY3.C,1)  IndexOptions=Select all,Index vector (dialog)  Indices=4:6,1:[N+4]  OutputSizes=1,1
  Step : Step  Time=2  SampleTime=0
  Sum1 : Sum  Inputs=|+-
  Sum2 : Sum  Inputs=|++
  Sum3 : Sum  Inputs=|+-
  Switch : Switch  Criteria=u2 > Threshold  SaturateOnIntegerOverflow=off  InputSameDT=off
  Switch1 : Switch  Criteria=u2 > Threshold  SaturateOnIntegerOverflow=off  InputSameDT=off
  Out2 : Outport  PortDimensions=[6,[N+4]]
  wires:
  Sum3/1 -> Switch1/1
  Int_DQNc_Mat2/1(Zpnz) -> Mult_DQNc_Mat2/2(Ydcpnz_c)  "xd"
  Gain4/1 -> Sum1/1, Switch/3
  [Ilow_dqn_inv] -> Mult_DQNc_Mat4/2(Ydcpnz_c)
  [Iup_dqn_inv] -> Mult_DQNc_Mat3/2(Ydcpnz_c)
  [Uref_dqn_inv] -> Switch1/3, Sum3/1
  Mult_DQNc_Mat1/1(Zdcpnz_c) -> Selector10/1
  Int_DQNc_Mat1/1(Zpnz) -> Mult_DQNc_Mat1/2(Ydcpnz_c)  "xd"
  Selector10/1 -> Mux13/1
  Mult_DQNc_Mat2/1(Zdcpnz_c) -> Selector11/1
  Gain7/1 -> Int_DQNc_Mat1/1(Xpnz)
  [Iup_dqn_inv] -> Sum2/1
  Switch/1 -> Add3/1
  Selector11/1 -> Mux13/2
  Gain15/1 -> Mult_DQNc_Mat2/1(Xdcpnz_c), Mult_DQNc_Mat4/1(Xdcpnz_c)
  [Ilow_dqn_inv] -> Sum2/2
  Mult_DQNc_Mat4/1(Zdcpnz_c) -> Gain1/1  "xd"
  Gain1/1 -> Int_DQNc_Mat2/1(Xpnz)
  [wtdq_inv] -> Circulating current suppression2/2(wt)
  Constant14/1 -> Add3/2
  Mult_DQNc_Mat3/1(Zdcpnz_c) -> Gain7/1  "xd"
  Gain6/1 -> Mult_DQNc_Mat1/1(Xdcpnz_c), Mult_DQNc_Mat3/1(Xdcpnz_c)
  Constant16/1 -> Add4/2
  [Uref_dqn_inv] -> Gain4/1
  Sum2/1 -> Circulating current suppression2/1(I_arm)
  Circulating current suppression2/2(-2Uref_dq0) -> Sum1/2, Sum3/2
  Add3/1 -> Gain6/1
  Switch1/1 -> Add4/1
  Add4/1 -> Gain15/1
  Sum1/1 -> Switch/1
  Step/1 -> Switch/2, Switch1/2
  Mux13/1 -> Out2/1

== system P2PHVDCMMC/Subsystem4/ACrec ==
  Add3 : Sum
  Add4 : Sum
  Circulating current suppression2 : Subsystem  VariantControl=Variant1
  Constant14 : Constant  Value="complex([[0 0; 0  0; 1 0 ],[zeros(3,N+2)]])"
  Constant16 : Constant  Value="complex([[0 0; 0  0; 1 0 ],[zeros(3,N+2)]])"
  Delay One Step2 : Delay  Commented=on  DelayLength=1  SampleTime=2e-5
  Gain1 : Gain  Gain=1/(C_PM / Nb_PM)
  Gain15 : Gain  Gain=0.5
  Gain4 : Gain  Gain=-1
  Gain6 : Gain  Gain=0.5
  Gain7 : Gain  Gain=1/(C_PM / Nb_PM)
  Int_DQNc_Mat1 : MATLAB Function  AncestorBlock=DQN_Lib/Int_DQNc_Mat  TreatAsAtomicUnit=on  SystemSampleTime=Ts_dqn  mask{N=7+N, dt=2e-5, w=Ws, InitInt=0*[0.8; 0.6; -0.33], swFeed=off, R=1, iL=1}
      mask prompts: N "Order number:"; dt "Time step (s):"; w "Angular frequency (1/rad):"; InitInt "Initial conditions DC [3x1]:"; swFeed "Enable feedback"; R "Feedback parameter (Kr {abc}):"; iL "Feedback parameter (Ki {abc}):"
  Int_DQNc_Mat2 : MATLAB Function  AncestorBlock=DQN_Lib/Int_DQNc_Mat  TreatAsAtomicUnit=on  SystemSampleTime=Ts_dqn  mask{N=7+N, dt=2e-5, w=Ws, InitInt=0*[0.8; 0.6; -0.33], swFeed=off, R=1, iL=1}
      mask prompts: N "Order number:"; dt "Time step (s):"; w "Angular frequency (1/rad):"; InitInt "Initial conditions DC [3x1]:"; swFeed "Enable feedback"; R "Feedback parameter (Kr {abc}):"; iL "Feedback parameter (Ki {abc}):"
  Mult_DQNc_Mat1 : MATLAB Function  AncestorBlock=DQN_Lib/Mult_DQNc_Mat  TreatAsAtomicUnit=on  SystemSampleTime=Ts_dqn  mask{N=7+N, HrmDbl=on}
      mask prompts: N "Harmonic order:"; HrmDbl "Double Harmonic"
  Mult_DQNc_Mat2 : MATLAB Function  AncestorBlock=DQN_Lib/Mult_DQNc_Mat  TreatAsAtomicUnit=on  SystemSampleTime=Ts_dqn  mask{N=7+N, HrmDbl=on}
      mask prompts: N "Harmonic order:"; HrmDbl "Double Harmonic"
  Mult_DQNc_Mat3 : MATLAB Function  AncestorBlock=DQN_Lib/Mult_DQNc_Mat  TreatAsAtomicUnit=on  SystemSampleTime=Ts_dqn  mask{N=3+N, HrmDbl=on}
      mask prompts: N "Harmonic order:"; HrmDbl "Double Harmonic"
  Mult_DQNc_Mat4 : MATLAB Function  AncestorBlock=DQN_Lib/Mult_DQNc_Mat  TreatAsAtomicUnit=on  SystemSampleTime=Ts_dqn  mask{N=3+N, HrmDbl=on}
      mask prompts: N "Harmonic order:"; HrmDbl "Double Harmonic"
  Mux13 : Concatenate  Mode=Multidimensional array
  Rate Transition1 : RateTransition  OutPortSampleTime=Ts_Power
  Selector10 : Selector  NumberOfDimensions=2  InputPortWidth=size(SY3.C,1)  IndexOptions=Select all,Index vector (dialog)  Indices=4:6,1:[N+4]  OutputSizes=1,1
  Selector11 : Selector  NumberOfDimensions=2  InputPortWidth=size(SY3.C,1)  IndexOptions=Select all,Index vector (dialog)  Indices=4:6,1:[N+4]  OutputSizes=1,1
  Step : Step  Time=2  SampleTime=0
  Sum1 : Sum  Inputs=|+-
  Sum2 : Sum  Inputs=|++
  Sum3 : Sum  Inputs=|+-
  Switch : Switch  Criteria=u2 > Threshold  SaturateOnIntegerOverflow=off  InputSameDT=off
  Switch1 : Switch  Criteria=u2 > Threshold  SaturateOnIntegerOverflow=off  InputSameDT=off
  Out2 : Outport  PortDimensions=[6,[N+4]]
  wires:
  Sum1/1 -> Switch/1
  Add4/1 -> Gain15/1
  Switch1/1 -> Add4/1
  Add3/1 -> Gain6/1
  Circulating current suppression2/2(-2Uref_dq0) -> Sum3/2, Sum1/2
  Sum2/1 -> Circulating current suppression2/1(I_arm)
  [Uref_dqn_rec] -> Gain4/1
  Constant16/1 -> Add4/2
  Gain6/1 -> Mult_DQNc_Mat3/1(Xdcpnz_c), Mult_DQNc_Mat1/1(Xdcpnz_c)
  Mult_DQNc_Mat3/1(Zdcpnz_c) -> Gain7/1  "xd"
  Constant14/1 -> Add3/2
  [wtdq_rec] -> Circulating current suppression2/2(wt)
  Gain1/1 -> Int_DQNc_Mat2/1(Xpnz)
  Mult_DQNc_Mat4/1(Zdcpnz_c) -> Gain1/1  "xd"
  [Ilow_dqn_rec] -> Sum2/2
  Gain15/1 -> Mult_DQNc_Mat4/1(Xdcpnz_c), Mult_DQNc_Mat2/1(Xdcpnz_c)
  Selector11/1 -> Mux13/2
  Switch/1 -> Add3/1
  [Iup_dqn_rec] -> Sum2/1
  Gain7/1 -> Int_DQNc_Mat1/1(Xpnz)
  Mult_DQNc_Mat2/1(Zdcpnz_c) -> Selector11/1
  Selector10/1 -> Mux13/1
  Int_DQNc_Mat1/1(Zpnz) -> Mult_DQNc_Mat1/2(Ydcpnz_c)  "xd"
  Mult_DQNc_Mat1/1(Zdcpnz_c) -> Selector10/1
  [Uref_dqn_rec] -> Sum3/1, Switch1/3
  Step/1 -> Rate Transition1/1
  [Iup_dqn_rec] -> Mult_DQNc_Mat3/2(Ydcpnz_c)
  [Ilow_dqn_rec] -> Mult_DQNc_Mat4/2(Ydcpnz_c)
  Gain4/1 -> Switch/3, Sum1/1
  Int_DQNc_Mat2/1(Zpnz) -> Mult_DQNc_Mat2/2(Ydcpnz_c)  "xd"
  Sum3/1 -> Switch1/1
  Rate Transition1/1 -> Switch1/2, Switch/2
  Mux13/1 -> Out2/1

== system P2PHVDCMMC/Subsystem4/Subsystem ==
  note: Vsec_inv
  In2 : Inport
  DQn->ABC1 : MATLAB Function  TreatAsAtomicUnit=on  SystemSampleTime=Ts_Power  mask{N=N+3}
      mask prompts: N "Harmonic order:"
  DQn->ABC10 : MATLAB Function  TreatAsAtomicUnit=on  SystemSampleTime=Ts_Power  mask{N=N+3}
      mask prompts: N "Harmonic order:"
  DQn->ABC11 : MATLAB Function  TreatAsAtomicUnit=on  SystemSampleTime=Ts_Power  mask{N=N+3}
      mask prompts: N "Harmonic order:"
  DQn->ABC12 : MATLAB Function  TreatAsAtomicUnit=on  SystemSampleTime=Ts_Power  mask{N=N+3}
      mask prompts: N "Harmonic order:"
  DQn->ABC14 : MATLAB Function  TreatAsAtomicUnit=on  SystemSampleTime=Ts_Power  mask{N=N+3}
      mask prompts: N "Harmonic order:"
  DQn->ABC17 : MATLAB Function  TreatAsAtomicUnit=on  SystemSampleTime=Ts_Power  mask{N=N+3}
      mask prompts: N "Harmonic order:"
  DQn->ABC18 : MATLAB Function  TreatAsAtomicUnit=on  SystemSampleTime=Ts_Power  mask{N=N+3}
      mask prompts: N "Harmonic order:"
  DQn->ABC2 : MATLAB Function  TreatAsAtomicUnit=on  SystemSampleTime=Ts_Power  mask{N=N+3}
      mask prompts: N "Harmonic order:"
  DQn->ABC8 : MATLAB Function  TreatAsAtomicUnit=on  SystemSampleTime=Ts_Power  mask{N=N+3}
      mask prompts: N "Harmonic order:"
  Mux{2..6,9} (6 alike) : Mux  Inputs=2
  Selector1 : Selector  NumberOfDimensions=2  InputPortWidth=size(S.C,1)  IndexOptions=Index vector (dialog),Select all  Indices=37:39,1  OutputSizes=1,1
  Selector17 : Selector  NumberOfDimensions=2  InputPortWidth=size(S.C,1)  IndexOptions=Index vector (dialog),Select all  Indices=22:24,1  OutputSizes=1,1
  Selector19 : Selector  NumberOfDimensions=2  InputPortWidth=size(S.C,1)  IndexOptions=Index vector (dialog),Select all  Indices=25:27,1  OutputSizes=1,1
  Selector22 : Selector  NumberOfDimensions=2  InputPortWidth=size(S.C,1)  IndexOptions=Index vector (dialog),Select all  Indices=4:6,1  OutputSizes=1,1
  Selector28 : Selector  NumberOfDimensions=2  InputPortWidth=size(S.C,1)  IndexOptions=Index vector (dialog),Select all  Indices=16:18,1  OutputSizes=1,1
  Selector29 : Selector  NumberOfDimensions=2  InputPortWidth=size(S.C,1)  IndexOptions=Index vector (dialog),Select all  Indices=19:21,1  OutputSizes=1,1
  Selector3 : Selector  NumberOfDimensions=2  InputPortWidth=size(S.C,1)  IndexOptions=Index vector (dialog),Select all  Indices=40:42,1  OutputSizes=1,1
  Selector32 : Selector  NumberOfDimensions=2  InputPortWidth=size(S.C,1)  IndexOptions=Index vector (dialog),Select all  Indices=13:15,1  OutputSizes=1,1
  Selector35 : Selector  NumberOfDimensions=2  InputPortWidth=size(S.C,1)  IndexOptions=Index vector (dialog),Select all  Indices=28:30,1  OutputSizes=1,1
  tag scope: Ilow_dqn_inv=global, Ilow_dqn_rec=global, Isec_dqn_inv=global, Isec_dqn_rec=global, Iup_dqn_inv=global, Iup_dqn_rec=global, Vdc_dqn=global, Vdcdqn=global, Vesc_in_DQn=global, Vsc_rec_DQn=global, Vsec_dqn_inv=global, Vsec_dqn_rec=global
  wires:
  [Isec] -> Mux5/1
  Selector35/1 -> [Ilow_dqn_rec], DQn->ABC18/1(Xdcpnz_c)
  In2/1 -> Selector22/1, Selector32/1, Selector1/1, Selector3/1, Selector35/1, Selector19/1, Selector17/1, Selector29/1, Selector28/1
  Selector28/1 -> [Vsec_dqn_inv], DQn->ABC17/1(Xdcpnz_c)
  Selector32/1 -> [Vsec_dqn_rec], DQn->ABC11/1(Xdcpnz_c)
  [wt0] -> DQn->ABC1/2(tho), DQn->ABC2/2(tho), DQn->ABC18/2(tho), DQn->ABC10/2(tho), DQn->ABC8/2(tho), DQn->ABC12/2(tho), DQn->ABC17/2(tho), DQn->ABC11/2(tho), DQn->ABC14/2(tho)  "theta"
  Selector17/1 -> [Ilow_dqn_inv], DQn->ABC8/1(Xdcpnz_c)
  Selector22/1 -> [Vdcdqn], DQn->ABC14/1(Xdcpnz_c)
  DQn->ABC2/1(Xabc) -> Mux9/2  "Mac_EMT"
  Selector1/1 -> [Isec_dqn_rec], DQn->ABC1/1(Xdcpnz_c)
  Selector19/1 -> [Iup_dqn_rec], DQn->ABC10/1(Xdcpnz_c)
  DQn->ABC10/1(Xabc) -> Mux4/2  "Mac_EMT"
  Selector3/1 -> [Isec_dqn_inv], DQn->ABC2/1(Xdcpnz_c)
  [Isec_inv] -> Mux9/1
  Selector29/1 -> [Iup_dqn_inv], DQn->ABC12/1(Xdcpnz_c)
  DQn->ABC17/1(Xabc) -> [Vesc_in_DQn]  "Mac_EMT"
  DQn->ABC1/1(Xabc) -> Mux5/2  "Mac_EMT"
  DQn->ABC8/1(Xabc) -> Mux3/2  "Mac_EMT"
  DQn->ABC11/1(Xabc) -> [Vsc_rec_DQn]  "Mac_EMT"
  DQn->ABC14/1(Xabc) -> [Vdc_dqn]  "Mac_EMT"
  DQn->ABC18/1(Xabc) -> Mux6/2  "Mac_EMT"
  DQn->ABC12/1(Xabc) -> Mux2/2  "Mac_EMT"
  [Iupmc_inv] -> Mux2/1
  [Ilowmc_inv] -> Mux3/1
  [Ilowmc] -> Mux6/1
  [Iupmc] -> Mux4/1

== system P2PHVDCMMC/Control _DQn_inv/Current Regulator (Ireg)2/PI regulator with anti-windup D ==
  note: Anti-windup mechanism: Method of conditionnal integration
      |
      | The integration is suspended if saturation occurs and the
      | control error is of the same sign as the control signal.
      |
      | [1] L.Rundqwist, "Anti-Reset Windup for PID Controllers," Ph.D. Thesis TRFT-1033,
      | Departement of Automatic Control, Lund Institute of Technology, Lund, Sweeden, 1991.
  Error : Inport  SampleTime=Ts
  Compare To Zero : simulink/Logic and Bit Operations/Compare To Zero  relop=>  OutDataTypeStr=uint8  ZeroCross=off
  Compare To Zero1 : simulink/Logic and Bit Operations/Compare To Zero  relop=<  OutDataTypeStr=uint8  ZeroCross=off
  Constant : Constant  Value=0
  Constant1 : Constant  Value=UpperLimit
  Constant3 : Constant  Value=LowerLimit
  Discrete-Time Integrator : DiscreteIntegrator  IntegratorMethod=Integration: Trapezoidal  InitialCondition=Init  SampleTime=Ts  LimitOutput=on  UpperSaturationLimit=UpperLimit  LowerSaturationLimit=LowerLimit  ShowStatePort=on  ICPrevOutput=DiscIntNeverNeededParam  ICPrevScaledInput=DiscIntNeverNeededParam
  Kp4 : Gain  Gain=Kp  SaturateOnIntegerOverflow=on  SampleTime=Ts  OutDataTypeStr=Inherit: Same as input  ParamDataTypeStr=Inherit: Same as input
  Kp5 : Gain  Gain=Ki  SaturateOnIntegerOverflow=on  SampleTime=Ts  OutDataTypeStr=Inherit: Same as input  ParamDataTypeStr=Inherit: Same as input
  Logical Operator : Logic  AllPortsSameDT=off  OutDataTypeStr=boolean
  Logical Operator1 : Logic  AllPortsSameDT=off  OutDataTypeStr=boolean
  Logical Operator2 : Logic  Operator=OR  AllPortsSameDT=off  OutDataTypeStr=boolean
  Relational Operator : RelationalOperator  OutDataTypeStr=boolean  InputSameDT=off
  Relational Operator1 : RelationalOperator  Operator=<=  OutDataTypeStr=boolean  InputSameDT=off
  Saturation2 : Saturate  UpperLimit=UpperLimit  LowerLimit=LowerLimit  SampleTime=Ts
  Sum1 : Sum  InputSameDT=on  SaturateOnIntegerOverflow=on  SampleTime=Ts  OutDataTypeStr=Inherit: Same as first input
  Sum6 : Sum  InputSameDT=on  SaturateOnIntegerOverflow=on  SampleTime=Ts  OutDataTypeStr=Inherit: Same as first input
  Switch : Switch  Criteria=u2 > Threshold  SaturateOnIntegerOverflow=off  InputSameDT=off
  Zero-Order Hold : ZeroOrderHold  SampleTime=Ts
  Out : Outport  SampleTime=Ts  InitialOutput=0
  wires:
  Constant/1 -> Switch/1
  Zero-Order Hold/1 -> Sum1/2, Sum6/1
  Discrete-Time Integrator/State -> Sum1/1
  Sum1/1 -> Relational Operator1/1, Relational Operator/1
  Logical Operator2/1 -> Switch/2
  Relational Operator/1 -> Logical Operator/1  "UpperLimit_is_Reached"
  Relational Operator1/1 -> Logical Operator1/1  "LowerLimit_Is_Reached"
  Constant1/1 -> Relational Operator/2
  Constant3/1 -> Relational Operator1/2
  Compare To Zero/1 -> Logical Operator/2  "Error_is_positive"
  Logical Operator/1 -> Logical Operator2/1
  Logical Operator1/1 -> Logical Operator2/2
  Compare To Zero1/1 -> Logical Operator1/2  "Error_is_negative"
  Error/1 -> Compare To Zero1/1, Compare To Zero/1, Kp4/1, Kp5/1
  Sum6/1 -> Saturation2/1
  Kp4/1 -> Zero-Order Hold/1
  Discrete-Time Integrator/1 -> Sum6/2
  Saturation2/1 -> Out/1
  Switch/1 -> Discrete-Time Integrator/1
  Kp5/1 -> Switch/3
